simulink model "real_time_diagram"  (R2021a)
settings: Solver=ode45  StartTime=0.0  StopTime=10  FixedStep=0.005  RelTol=1e-3
undefined symbols (not defined in the file): K, National_Instruments, PCI, Ts, wc, x_d
libraries: sldrtlib x2, simulink_extras x1
settings Model: SimulationMode=external  ExtModeTrigDuration=200000  Creator=magudelo  LastModifiedBy=martijndebeuf
settings SolverCC: AlgebraicLoopSolver=TrustRegion  InsertRTBMode=Always
settings DataIOCC: LimitDataPoints=on  SaveFormat=Array  SignalLoggingSaveFormat=ModelDataLogs  ReturnWorkspaceOutputs=off
settings OptimizationCC: ExpressionDepthLimit=2147483647
settings DebuggingCC: UnderspecifiedInitializationDetection=Classic  MergeDetectMultiDrivingBlocksExec=none  SolverPrmCheckMsg=warning  FcnCallInpInsideContextMsg=warning  StateNameClashWarn=warning  SFUnexpectedBacktrackingDiag=warning  SFNoUnconditionalDefaultTransitionDiag=warning  SFExecutionAtInitializationDiag=none  SFMachineParentedDataDiag=warning  ArithmeticOperatorsInVariantConditions=warning
settings ModelReferenceCC: PropagateSignalLabelsOutOfModel=off
settings SFSimCC: SimUseLocalCustomCode=off  CustomCodeUndefinedFunction=UseInterfaceOnly
settings RTWCC: Description=Simulink Desktop Real-Time  SystemTargetFile=sldrt.tlc  TemplateMakefile=sldrt.tmf  RTWUseLocalCustomCode=off  RTWCompilerOptimization=on
settings CodeAppCC: MaxIdLength=95  StateflowObjectComments=on
settings TargetCC: TargetPreCompLibLocation=C:\Program Files\MATLAB\R2018a\toolbox\sldrt\lib\win64
settings ConfigComp: CovMetricSettings=dw  CovSaveCumulativeToWorkspaceVar=on  CovSaveSingleToWorkspaceVar=on  CovExternalEMLEnable=off

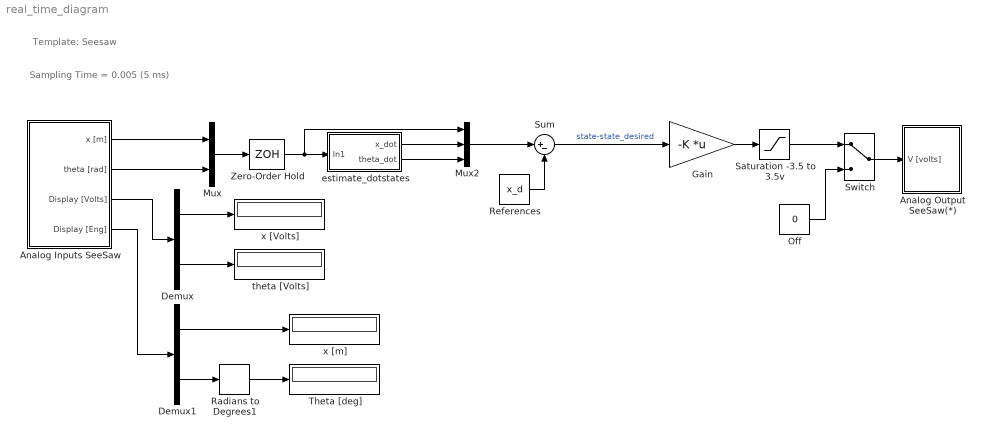
== system real_time_diagram ==
  note: Template: Seesaw
  note: Sampling Time = 0.005 (5 ms)
  Analog Inputs SeeSaw : Subsystem  mask(Analog Inputs. SeeSaw){v2m=0.1033, offset_x=0, v2r=-0.0827, offset_theta=-5.56}
      mask prompts: v2m "F_x = Conversion factor from Volts to Meters:"; offset_x "Off_x = Offset for Cart Position [Volts] :"; v2r "F_theta = Conversion Factor From Volts to Radians :"; offset_theta "Off_theta = Offset for the angle of the SeeSaw [Volts] :"
      mask help:
      | Remember:
      |    Cart Position (x)                     => channel ACH0
      |    Angle of the SeeSaw (theta) => channel ACH1
      |
      |   Cart Position [m] = F_x *  ( Cart Position [v] + off_x )
      |   Angle of the SeeSaw [rad] = F_theta *  ( Angle of the SeeSaw [v] + off_theta )
  "Analog Output SeeSaw(*) " : Subsystem  mask(Analog Output - SeeSaw){}
      mask help:
      | Remember
      |    AO 0 => Power Amplifier + Motor
  Demux : Demux  Outputs=2
  Demux1 : Demux  Outputs=2
  Gain : Gain  Gain=-K  Multiplication=Matrix(K*u) (u vector)
  Mux : Mux  Inputs=2
  Mux2 : Mux  Inputs=3
  Off : Constant  Value=0
  Radians to Degrees1 : simulink_extras/Transformations/Radians to Degrees
  References : Constant  Value=x_d
  Saturation -3.5 to 3.5v : Saturate  UpperLimit=3.5  LowerLimit=-3.5
  Sum : Sum  Inputs=|+-
  "Switch  " : ManualSwitch
  Theta [deg] : Display
      settings: SampleTime=0.25
  Zero-Order Hold : ZeroOrderHold  SampleTime=-1
  estimate_dotstates : Subsystem
  theta [Volts] : Display
      settings: SampleTime=0.25
  x [Volts] : Display
      settings: SampleTime=0.25
  x [m] : Display
      settings: SampleTime=0.25
  wires:
  Demux/1 -> x [Volts]/1
  Demux/2 -> theta [Volts]/1
  Analog Inputs SeeSaw/3(Display [Volts]) -> Demux/1
  Analog Inputs SeeSaw/4(Display [Eng]) -> Demux1/1
  Off/1 -> "Switch  "/2
  "Switch  "/1 -> "Analog Output SeeSaw(*) "/1(V [volts])
  Demux1/1 -> x [m]/1
  Demux1/2 -> Radians to Degrees1/1
  Radians to Degrees1/1 -> Theta [deg]/1
  Saturation -3.5 to 3.5v/1 -> "Switch  "/1
  estimate_dotstates/1(x_dot) -> Mux2/2
  Sum/1 -> Gain/1  "state-state_desired"
  Mux2/1 -> Sum/1
  References/1 -> Sum/2
  Analog Inputs SeeSaw/1(x [m]) -> Mux/1
  Analog Inputs SeeSaw/2(theta [rad]) -> Mux/2
  Gain/1 -> Saturation -3.5 to 3.5v/1
  estimate_dotstates/2(theta_dot) -> Mux2/3
  Mux/1 -> Zero-Order Hold/1
  Zero-Order Hold/1 -> Mux2/1, estimate_dotstates/1(In1)

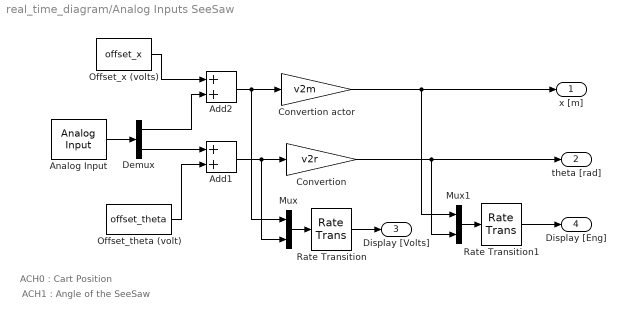
== system real_time_diagram/Analog Inputs SeeSaw ==
  note: ACH0 : Cart Position
  note: ACH1 : Angle of the SeeSaw
  Add1 : Sum
  Add2 : Sum
  Analog Input : sldrtlib/Analog Input  SampleTime=0.005  MaxMissedTicks=10  ShowMissedTicks=off  YieldWhenWaiting=off  DrvName=National_Instruments/PCI-6014  DrvAddress=4294967295  DrvOptions=[1 0 0 0 0 0]  Channels=[1 2]  RangeMode=1  VoltRange=1  DataType=1
      settings: AttributesFormatString=National Instruments\nPCI-6014 [auto]
  "Convertion " : Gain  Gain=v2r
  Convertion actor : Gain  Gain=v2m
  Demux : Demux  Outputs=2
  Mux : Mux  Inputs=2
  Mux1 : Mux  Inputs=2
  Offset_theta (volt) : Constant  Value=offset_theta
  Offset_x (volts) : Constant  Value=offset_x
  Rate Transition : RateTransition  OutPortSampleTime=0.25
  Rate Transition1 : RateTransition  OutPortSampleTime=0.25
  x [m] : Outport  VectorParamsAs1DForOutWhenUnconnected=off
  theta [rad] : Outport  Port=2  VectorParamsAs1DForOutWhenUnconnected=off
  Display [Volts] : Outport  Port=3  VectorParamsAs1DForOutWhenUnconnected=off
  Display [Eng] : Outport  Port=4  VectorParamsAs1DForOutWhenUnconnected=off
  wires:
  Analog Input/1 -> Demux/1
  Demux/1 -> Add2/2
  Add2/1 -> Convertion actor/1, Mux/1
  Offset_x (volts)/1 -> Add2/1
  Convertion actor/1 -> x [m]/1, Mux1/1
  Demux/2 -> Add1/1
  Offset_theta (volt)/1 -> Add1/2
  Add1/1 -> "Convertion "/1, Mux/2
  "Convertion "/1 -> theta [rad]/1, Mux1/2
  Rate Transition/1 -> Display [Volts]/1
  Mux/1 -> Rate Transition/1
  Mux1/1 -> Rate Transition1/1
  Rate Transition1/1 -> Display [Eng]/1

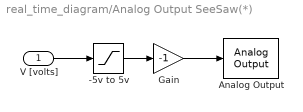
== system real_time_diagram/Analog Output SeeSaw(*)  ==
  V [volts] : Inport
  -5v to 5v : Saturate  UpperLimit=5  LowerLimit=-5
  Analog Output : sldrtlib/Analog Output  SampleTime=0.005  MaxMissedTicks=10  ShowMissedTicks=off  YieldWhenWaiting=off  DrvName=National_Instruments/PCI-6014  DrvAddress=4294967295  DrvOptions=[1 0 0 0 0 0]  Channels=1  RangeMode=1  VoltRange=1  InitialValue=0  FinalValue=0
      settings: AttributesFormatString=National Instruments\nPCI-6014 [auto]
  Gain : Gain  Gain=-1
  wires:
  Gain/1 -> Analog Output/1
  -5v to 5v/1 -> Gain/1
  V [volts]/1 -> -5v to 5v/1

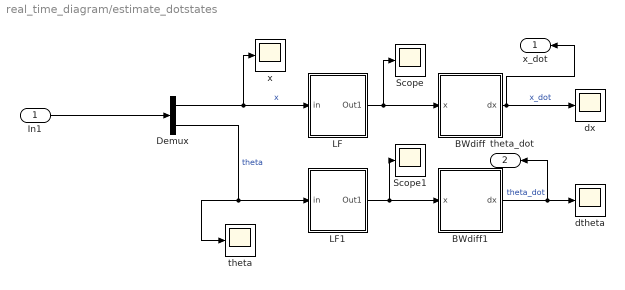
== system real_time_diagram/estimate_dotstates ==
  In1 : Inport
  BWdiff : Subsystem
  BWdiff1 : Subsystem
  Demux : Demux  Outputs=2
  LF : Subsystem
  LF1 : Subsystem
  Scope : Scope
  Scope1 : Scope
  dtheta : Scope
  dx : Scope
  theta : Scope
  x : Scope
  x_dot : Outport
  theta_dot : Outport  Port=2
  wires:
  LF1/1(Out1) -> Scope1/1, BWdiff1/1(x)
  Demux/2 -> LF1/1(in), theta/1  "theta"
  In1/1 -> Demux/1
  BWdiff1/1(dx) -> theta_dot/1, dtheta/1  "theta_dot"
  LF/1(Out1) -> Scope/1, BWdiff/1(x)
  BWdiff/1(dx) -> x_dot/1, dx/1  "x_dot"
  Demux/1 -> LF/1(in), x/1  "x"

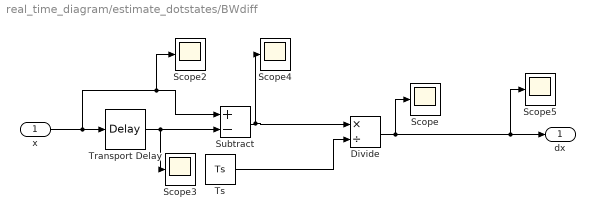
== system real_time_diagram/estimate_dotstates/BWdiff ==
  x : Inport
  Divide : Product  Inputs=*/
  Scope{,2..5} (5 alike) : Scope
  Subtract : Sum  Inputs=+-
  Transport Delay : TransportDelay  DelayTime=Ts
  Ts : Constant  Value=Ts
  dx : Outport
  wires:
  Transport Delay/1 -> Scope3/1, Subtract/2
  Ts/1 -> Divide/2
  x/1 -> Transport Delay/1, Scope2/1, Subtract/1
  Subtract/1 -> Divide/1, Scope4/1
  Divide/1 -> Scope5/1, dx/1, Scope/1

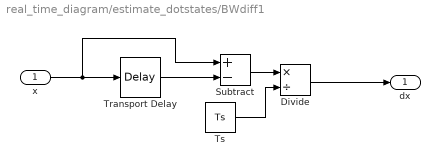
== system real_time_diagram/estimate_dotstates/BWdiff1 ==
  x : Inport
  Divide : Product  Inputs=*/
  Subtract : Sum  Inputs=+-
  Transport Delay : TransportDelay  DelayTime=Ts
  Ts : Constant  Value=Ts
  dx : Outport
  wires:
  Ts/1 -> Divide/2
  Subtract/1 -> Divide/1
  x/1 -> Transport Delay/1, Subtract/1
  Divide/1 -> dx/1
  Transport Delay/1 -> Subtract/2

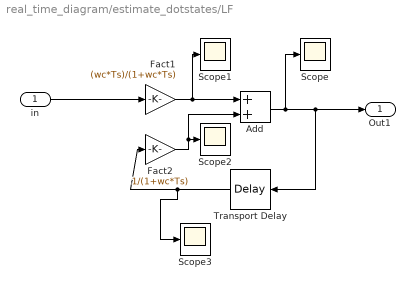
== system real_time_diagram/estimate_dotstates/LF ==
  in : Inport
  Add : Sum
  Fact1 : Gain  Gain=(wc*Ts)/(1+wc*Ts)
  Fact2 : Gain  Gain=1/(1+wc*Ts)
  Scope{,1..3} (4 alike) : Scope
  Transport Delay : TransportDelay  DelayTime=Ts
  Out1 : Outport
  wires:
  Fact2/1 -> Add/2, Scope2/1
  Fact1/1 -> Scope1/1, Add/1
  in/1 -> Fact1/1
  Add/1 -> Scope/1, Transport Delay/1, Out1/1
  Transport Delay/1 -> Scope3/1, Fact2/1

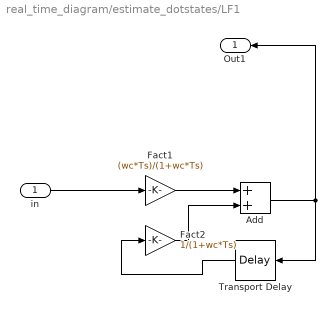
== system real_time_diagram/estimate_dotstates/LF1 ==
  in : Inport
  Add : Sum
  Fact1 : Gain  Gain=(wc*Ts)/(1+wc*Ts)
  Fact2 : Gain  Gain=1/(1+wc*Ts)
  Transport Delay : TransportDelay  DelayTime=Ts
  Out1 : Outport
  wires:
  Add/1 -> Transport Delay/1, Out1/1
  Fact2/1 -> Add/2
  Fact1/1 -> Add/1
  in/1 -> Fact1/1
  Transport Delay/1 -> Fact2/1
